simulink subsystem "SIGN_EXTEND_04_SS"  (R2022a)
settings: Solver=VariableStepAuto  StartTime=0.0  StopTime=10.0  RelTol=1e-3
libraries: hdlBasic x11
settings Model: Creator=sebas  LastModifiedBy=viktor

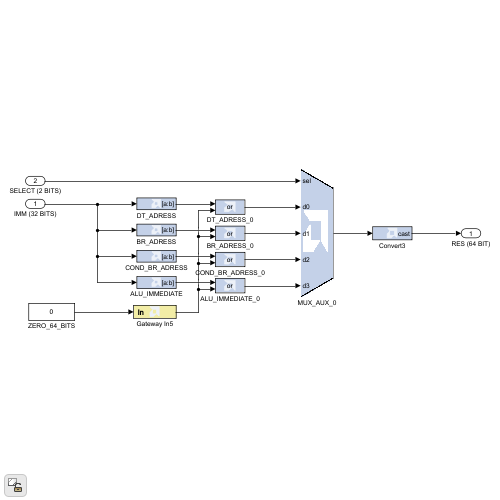
[thumbnail: Simulink's stored preview of the top-level diagram]
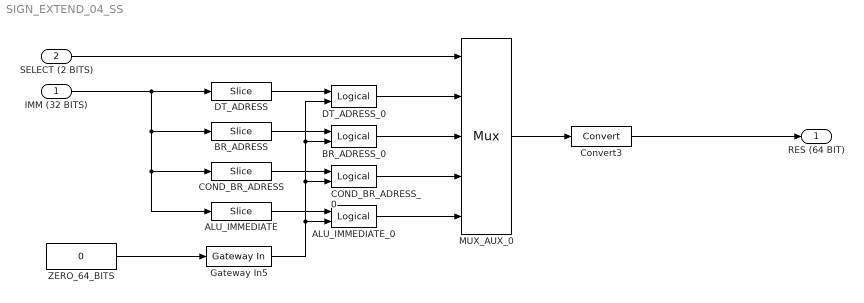
== system SIGN_EXTEND_04_SS ==
  IMM (32 BITS) : Inport
  SELECT (2 BITS) : Inport  Port=2
  ALU_IMMEDIATE : hdlBasic/Slice  nbits=16  boolean_output=off  mode=Two Bit Locations  bit1=21  base1=LSB of Input  bit0=10  base0=LSB of Input  XmcBlockStatus=1  maskContainerNames=group1  block_type=slice  block_config=sysgen:Slice_config
  ALU_IMMEDIATE_0 : hdlBasic/Logical  logical_function=OR  inputs=2  en=off  latency=0  precision=Full  arith_type=Unsigned  n_bits=16  bin_pt=0  align_bp=on  overflow=[]  quantization=[]  XmcBlockStatus=1  maskContainerNames=tabcontainer1  block_type=logical  block_config=sysgen:Logical_config
  BR_ADRESS : hdlBasic/Slice  nbits=16  boolean_output=off  mode=Two Bit Locations  bit1=25  base1=LSB of Input  bit0=0  base0=LSB of Input  XmcBlockStatus=1  maskContainerNames=group1  block_type=slice  block_config=sysgen:Slice_config
  BR_ADRESS_0 : hdlBasic/Logical  logical_function=OR  inputs=2  en=off  latency=0  precision=Full  arith_type=Unsigned  n_bits=16  bin_pt=0  align_bp=on  overflow=[]  quantization=[]  XmcBlockStatus=1  maskContainerNames=tabcontainer1  block_type=logical  block_config=sysgen:Logical_config
  COND_BR_ADRESS : hdlBasic/Slice  nbits=16  boolean_output=off  mode=Two Bit Locations  bit1=23  base1=LSB of Input  bit0=5  base0=LSB of Input  XmcBlockStatus=1  maskContainerNames=group1  block_type=slice  block_config=sysgen:Slice_config
  COND_BR_ADRESS_0 : hdlBasic/Logical  logical_function=OR  inputs=2  en=off  latency=0  precision=Full  arith_type=Unsigned  n_bits=16  bin_pt=0  align_bp=on  overflow=[]  quantization=[]  XmcBlockStatus=1  maskContainerNames=tabcontainer1  block_type=logical  block_config=sysgen:Logical_config
  Convert3 : hdlBasic/Convert  gui_display_data_type=Fixed-point  arith_type=Unsigned  n_bits=64  bin_pt=0  float_type=Single  exp_bits=8  fraction_bits=24  quantization=Truncate  overflow=Wrap  en=off  latency=0  pipeline=off  XmcBlockStatus=1  maskContainerNames=group2  block_type=convert  block_config=sysgen:Convert_config  block_width=595  block_height=885
  DT_ADRESS : hdlBasic/Slice  nbits=16  boolean_output=off  mode=Two Bit Locations  bit1=20  base1=LSB of Input  bit0=12  base0=LSB of Input  XmcBlockStatus=1  maskContainerNames=group1  block_type=slice  block_config=sysgen:Slice_config
  DT_ADRESS_0 : hdlBasic/Logical  logical_function=OR  inputs=2  en=off  latency=0  precision=Full  arith_type=Unsigned  n_bits=16  bin_pt=0  align_bp=on  overflow=[]  quantization=[]  XmcBlockStatus=1  maskContainerNames=tabcontainer1  block_type=logical  block_config=sysgen:Logical_config
  Gateway In5 : hdlBasic/Gateway In  gui_display_data_type=Fixed-point  arith_type=Unsigned  n_bits=64  bin_pt=0  preci_type=Single  exp_width=8  frac_width=24  rows=1  columns=1  quantization="Round  (unbiased: +/- Inf)"  overflow=Saturate  period=1  UseAsADC=off  ADCChannel='1'  interface=None  automatic_assignment=on  address_offset=hex2dec('00')  intf_name=''  intf_description=''  default_value=0  timing_constraint=None  locs_specified=off  LOCs={}  io_standard={}  inherit_from_input=off  hdl_port=on  XmcBlockStatus=1  maskContainerNames=group4  block_type=gatewayin  block_config=sysgen:gateway_in_config  block_width_w=590  block_height_w=620  block_width=640  block_height=850
  MUX_AUX_0 : hdlBasic/Mux  inputs=4  en=off  latency=0  precision=Full  arith_type=Unsigned  n_bits=16  bin_pt=14  quantization=Truncate  overflow=Wrap  XmcBlockStatus=1  maskContainerNames=tabcontainer1  block_type=mux  block_config=sysgen:Mux_config
  ZERO_64_BITS : Constant  Value=0
  RES (64 BIT) : Outport
  wires:
  Gateway In5/1 -> DT_ADRESS_0/2, BR_ADRESS_0/2, COND_BR_ADRESS_0/2, ALU_IMMEDIATE_0/2
  SELECT (2 BITS)/1 -> MUX_AUX_0/1
  BR_ADRESS_0/1 -> MUX_AUX_0/3
  ZERO_64_BITS/1 -> Gateway In5/1
  IMM (32 BITS)/1 -> DT_ADRESS/1, BR_ADRESS/1, COND_BR_ADRESS/1, ALU_IMMEDIATE/1
  ALU_IMMEDIATE_0/1 -> MUX_AUX_0/5
  COND_BR_ADRESS_0/1 -> MUX_AUX_0/4
  DT_ADRESS_0/1 -> MUX_AUX_0/2
  BR_ADRESS/1 -> BR_ADRESS_0/1
  Convert3/1 -> RES (64 BIT)/1
  MUX_AUX_0/1 -> Convert3/1
  COND_BR_ADRESS/1 -> COND_BR_ADRESS_0/1
  ALU_IMMEDIATE/1 -> ALU_IMMEDIATE_0/1
  DT_ADRESS/1 -> DT_ADRESS_0/1
